simulink model "FreqBandInvest"  (R2018a)
settings: Solver=VariableStepAuto  StartTime=0.0  StopTime=0.01  RelTol=1e-3
values from neighbouring files (symbols this model uses):
  G1 = 10^(G1dB/10)    (= 20323.5701094)    [SimVar.m]
  G2 = 10^(G2dB/10)    (= 358921.934645)    [SimVar.m]
  T = 1/Fs    (= 5e-05)    [SimVar.m]
undefined symbols (not defined in the file or in its folder): fdesignblkfcn, gcbh, get
libraries: dspsrcs4 x1, dspxfrm3 x1, dspobslib x1
settings Model: Creator=Daniel  LastModifiedBy=Daniel

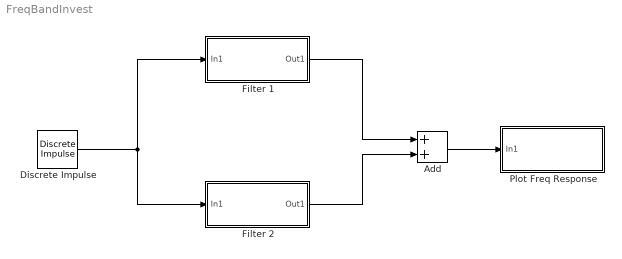
== system FreqBandInvest ==
  Add : Sum
  Discrete Impulse : dspsrcs4/Discrete  Impulse  Delay=0  SampleTime=T  FrameSample=128  OutputFrames=off  dataType=double  isSigned=on  wordLen=16  udDataType=sfix(16)  fracBitsMode=Best precision  numFracBits=15  OutDataTypeStr=double  LastOutDataTypeStr=double
  Filter 1 : Subsystem
  Filter 2 : Subsystem
  Plot Freq Response : Subsystem
  wires:
  Discrete Impulse/1 -> Filter 2/1(In1), Filter 1/1(In1)
  Add/1 -> Plot Freq Response/1(In1)
  Filter 1/1(Out1) -> Add/1
  Filter 2/1(Out1) -> Add/2

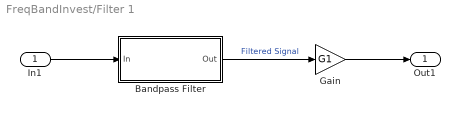
== system FreqBandInvest/Filter 1 ==
  In1 : Inport
  Bandpass Filter : Subsystem  DialogController=fdesignblkfcn  InitFcn=fdesignblkfcn(gcbh, {'InitFcn'});  mask(Bandpass Filter){}
      mask help: Design a bandpass filter
      settings: CopyFcn=fdesignblkfcn(gcbh, {'CopyFcn'});
      mask Help: helpview(mapfilelocation('dsp'), 'dspbandpassfilter');
      mask Display: disp('Bandpass');
  Gain : Gain  Gain=G1
  Out1 : Outport
  wires:
  Bandpass Filter/1(Out) -> Gain/1  "Filtered Signal"
  In1/1 -> Bandpass Filter/1(In)
  Gain/1 -> Out1/1

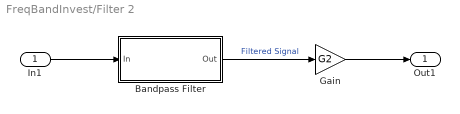
== system FreqBandInvest/Filter 2 ==
  In1 : Inport
  Bandpass Filter : Subsystem  DialogController=fdesignblkfcn  InitFcn=fdesignblkfcn(gcbh, {'InitFcn'});  mask(Bandpass Filter){}
      mask help: Design a bandpass filter
      settings: CopyFcn=fdesignblkfcn(gcbh, {'CopyFcn'});
      mask Help: helpview(mapfilelocation('dsp'), 'dspbandpassfilter');
      mask Display: disp('Bandpass');
  Gain : Gain  Gain=G2
  Out1 : Outport
  wires:
  Bandpass Filter/1(Out) -> Gain/1  "Filtered Signal"
  In1/1 -> Bandpass Filter/1(In)
  Gain/1 -> Out1/1

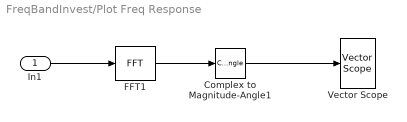
== system FreqBandInvest/Plot Freq Response ==
  In1 : Inport
  Complex to Magnitude-Angle1 : ComplexToMagnitudeAngle  Output=Magnitude
  FFT1 : dspxfrm3/FFT  FFTImplementation=Auto  CompMethod=Table lookup  TableOpt=NEW  TableOptActive=Speed  BitRevOrder=off  Normalize=off  InheritFFTLength=on  FFTLength=64  WrapInput=on  roundingMode=Floor  overflowMode=off  firstCoeffDataTypeStr=Inherit: Same word length as input  firstCoeffLastDataTypeStr=Inherit: Same word length as input  outputMin=[]  outputMax=[]
  Vector Scope : dspobslib/Vector Scope  ScopeProperties=off  Domain=Frequency  HorizSpan=1  DisplayProperties=off  AxisGrid=on  Memory=off  FrameNumber=off  AxisLegend=off  AxisZoom=off  OpenScopeAtSimStart=on  OpenScopeImmediately=off  FigPos=get(0,'defaultfigureposition')  AxisProperties=on  XUnits=Hertz  XRange=[0...Fs/2]  InheritXIncr=on  XIncr=1  XLabel=Samples  XLimit=Auto  XMin=0  XMax=1  XStart=0  YUnits=dB  YLabel=|Magnitude (dB)|  LineProperties=off  XAxisParamsVer=6.9
      settings: SourceProductName=DSP System Toolbox  SourceProductBaseCode=DS  YMin=0.0723692553519949  YMax=69.3188381671759
  wires:
  In1/1 -> FFT1/1
  FFT1/1 -> Complex to Magnitude-Angle1/1
  Complex to Magnitude-Angle1/1 -> Vector Scope/1

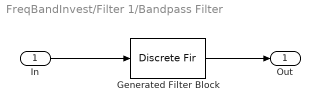
== system FreqBandInvest/Filter 1/Bandpass Filter ==
  In : Inport
  Generated Filter Block : DiscreteFir  Tag=BlockMethodSubSystem  Coefficients=[-6.22134684656821929e-07 -1.13803127657343925e-05 -6.88386174447548914e-05 -0.000253967523622427498 -0.000674852927024836759 -0.00138321611437446285 -0.00224615205437689834 -0.00287799561946159958 -0.00276478288326855413 -0.00160169913189871986 0.000353414578601418759 0.00224131512232661782 0.00305797231453537252 0.0023772015982347558 0.000770280234616252564 -0.000529027839585679898 -0.000563468590790226547 0.000557086889126886197 0.00174949556096017414 0.00192555029611151621 0.000982194780574025374 -0.000128810295873105728 -0.000345543385096612227 0.000460085962964390191 0.00138649354284238403 0.00145553707936558834 0.000626161778190072573 -0.000195711247121112009 -0.000153660688332653831 0.000638460939418158697 0.00125240560420236723 0.000993573560769381867 0.000166370232783301391 -0.000296934296058754552 9.02545340256092222e-05 0.000824819766955211869 0.00101745910882160458 0.000432607742948015283 -0.000250666566265708723 -0.000254756383560556605 0.000375210655804679829 0.000838268201188364557 0.000546319097839828441 -0.000171466041654512387 -0.000476090053441056841 -4.17435883611086972e-05 0.000550372287648921211 0.000528368533145709635 -0.000120512195016867402 -0.000635009309722105023 -0.000422415954668505747 0.00020428638829965716 0.000413116592135938799 -0.000108999680521119793 -0.000759374163185272746 -0.000769321483712461255 -0.000172031384687839234 0.000229435566692807346 -0.000130523332887852629 -0.0008574556021098415 -0.00108225819350876804 -0.000560797638061341424 1.59137300917482945e-06 -0.000167357505060817472 -0.000918202941862006372 -0.00134945192301835315 -0.000947380117339017571 -0.000256925687184635066 -0.000207572712342537845 -0.000924773256179438926 -0.00154499545210730425 -0.0013030654705771757 -0.000525149016806325574 -0.000239635683808835976 -0.000865706075121728006 -0.00164943140144713273 -0.00160388345451245411 -0.000783719210119303246 -0.000249764094114686723 -0.000723696809050329353 -0.00163635770377135756 -0.00182257973909121115 -0.00101762278312500271 -0.000234984245866535178 -0.000491645280086358484 -0.00148135369138719308 -0.00192483568008164959 -0.00120341123028480418 -0.000192010850813616256 -0.000172789965923526726 -0.00117472481882622756 -0.00188721337802484103 -0.00132214392012228025 -0.000119226114122434145 0.000227212538210782141 -0.000709601381017732581 -0.00168810266189821844 -0.00135813280073006685 -2.48918571033703834e-05 0.000685162712620597308 -9.72059754754235156e-05 -0.00131475396936935464 -0.0012928173798521026 8.94654598327188565e-05 0.00117784158381673931 0.000640798159544884397 -0.000770891250633719835 -0.00112488430410933715 0.000205220622413819666 0.00166488045333667819 0.00146993967623927028 -6.16298422594324755e-05 -0.000842591643983662034 0.00031473831611570724 0.00210257607389142433 0.00233376764695160692 0.000778243020106321741 -0.000455858600915155484 0.000403017571548850654 0.00244845119914128368 0.00317774903725895471 0.0017149320049159927 2.71371332816023155e-05 0.000454219136486538552 0.00264826842089186873 0.00392176733551483948 0.00268549335167518654 0.000582179642925996239 0.000457265203221198381 0.00266527096576633189 0.00450139560035541734 0.00363374991707076213 0.00118539453724563664 0.000397582835957589287 0.00245172875455694408 0.0048304673298412374 0.00447842084500495782 0.00180050584364714389 0.00027037548489263261 0.00198368676252074546 0.00484216455905152852 0.00514267490349157481 0.00238625823399260485 6.73386479935509052e-05 0.00123712322770924222 0.00446643428680088429 0.00554161419395732355 0.00289906631432766291 -0.000204049233068994372 0.000220204578073280617 0.00366525974041039112 0.00560723873909181169 0.00329758803960814636 -0.000537700933391743242 -0.0010581490277047636 0.00239885604856528937 0.00526380542706242783 0.0035358265753866803 -0.000914028162045346323 -0.00255407127749022328 0.00066922347615446659 0.00446629675043999468 0.00358391566531769462 -0.00130221661632914237 -0.00421162280403450297 -0.00151618469705966049 ...(+6736 chars)]  InputProcessing=Columns as channels (frame based)
  Out : Outport
  wires:
  In/1 -> Generated Filter Block/1
  Generated Filter Block/1 -> Out/1

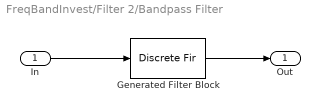
== system FreqBandInvest/Filter 2/Bandpass Filter ==
  In : Inport
  Generated Filter Block : DiscreteFir  Tag=BlockMethodSubSystem  Coefficients=[-3.39460949165395717e-06 1.3450936839256965e-05 -3.47685045710267847e-06 -6.23673651333002713e-05 9.42736662656093038e-05 8.68149844918313454e-05 -0.000321492861862216243 7.42688799067623215e-05 0.0005497663535907638 -0.000427751039768807257 -0.000648715942068820426 0.000801269067634722654 0.000814864650021221958 -0.001419893419875523 -0.00095720491948660634 0.00267918863363881404 6.69864647352538865e-05 -0.00358438632387772516 0.00203157449623721275 0.00229270016540182543 -0.0029315542756148563 0.000285551205655857243 0.000859048609545473834 -0.00063357268683205824 0.00146005434142504158 -0.00147970377780497924 -0.000835384755319627695 0.00209794252956948786 -0.000623005965591806317 -0.000319999264726182446 -0.000250705364319847178 -0.000324430942669484039 0.00147966888151390631 -0.00063969870960327844 -0.000647701851011092851 0.000210308048850518526 -3.53105490030912408e-06 0.00103623903000851 -0.00082686460101530487 -0.00059103060449822956 0.000609448351695299358 -8.39463278626153009e-06 0.000667241391010738386 -0.000843833918867074547 -0.000472913857123019685 0.000863011184082015156 -8.23734466595780768e-05 0.000354928110012965223 -0.000794159738940037534 -0.000296400534395932177 0.000990815273698306565 -0.000206904434880677987 0.00014010671661290525 -0.000727221672792353305 -0.000109997706078207835 0.00105865309718022036 -0.000374409617416737771 -1.97428333759443534e-06 -0.000637869758141187959 6.83338326967813172e-05 0.00108021814083011209 -0.000568443531816811148 -8.35490987902345335e-05 -0.000531603535252860655 0.000233545368361912792 0.00106486473930582858 -0.000781362094778957216 -0.000114698066690031852 -0.000409475710739667009 0.00038930805297684903 0.00101050626668713591 -0.00101580571716776793 -8.8514528333696142e-05 -0.000265633994023877949 0.000520640011103379232 0.000911196881272975353 -0.00125334316372880902 -1.01395617070277772e-06 -0.000114207267844458892 0.000624006276273571052 0.000773658461625423418 -0.00149158509188909282 0.000148032462349562507 4.86417455934120267e-05 0.000690316087440484387 0.000586150129934123374 -0.00171165906913728003 0.000373068742649320078 0.000201966002951985048 0.000704856618052459704 0.000362909413674368704 -0.00189736727021877949 0.000667694701011695667 0.000333047910917953099 0.000664478022441336688 0.000108071167633810481 -0.00203322633954709786 0.00103323481489765658 0.000421632263074327477 0.00056274189365219517 -0.000163339927538032846 -0.00210417293220937487 0.00146146167974254356 0.000449867128297573257 0.000396999200241856826 -0.000437630416999294954 -0.00209089813618481331 0.00194099252808805842 0.000389331219429741822 0.000172723145948520257 -0.000687194607197532509 -0.0019856062015907042 0.00244596154444125333 0.0002255001723221955 -9.42603572630244709e-05 -0.000898305693495389437 -0.00178175350700305267 0.00295935644665310535 -6.47274647532138379e-05 -0.000388069135390506261 -0.00104248494962693805 -0.0014818638275861276 0.00344893039558220741 -0.000489903232051619865 -0.000683044481746528792 -0.00110455458070272895 -0.00108966696006214023 0.00388745841774875518 -0.00106461847166327791 -0.000947110117354471874 -0.00105960386842996238 -0.000625499352313017257 0.00423858025583928773 -0.00178168915530105927 -0.00114364955301721953 -0.000901195978902788832 -0.000109627626810524735 0.00447433200325978234 -0.00263493864485979737 -0.00123469517981365318 -0.000621840554658022768 0.00043010487454228592 0.00456337764255932126 -0.00360603988166625445 -0.0011778029339457631 -0.000226518232776350484 0.000963370023933500757 0.00447808731431768685 -0.00467331673427785234 -0.000920961071934424977 0.000269670852772600431 0.0014427286989675942 0.00420749387156958612 -0.00579972319233663589 -0.000428819620008018818 0.000844560833419409282 0.00182894033706789989 0.00373830770185544893 -0.00694161453187636546 0.000338706214949100815 0.00145902157737988047 0.00208224312098644754 0.00307026482880855787 -0.00805389132705568861 0.00141839415647011888 0.00206625070378688939 ...(+6824 chars)]  InputProcessing=Columns as channels (frame based)
  Out : Outport
  wires:
  In/1 -> Generated Filter Block/1
  Generated Filter Block/1 -> Out/1
